simulink model "modelo"  (Simulink 10.0)
settings: Solver=VariableStepAuto  StartTime=0.0  StopTime=stop_time  FixedStep=stop_time/1000  RelTol=1e-5
values from neighbouring files (symbols this model uses):
  alfa1 = 1.4    [erro.m]    (also in natureza.m)
  alfa2 = val(2)    [erro.m]    (also in natureza.m = aux(2))
  delta1 = 3.1    [erro.m]    (also in natureza.m)
  delta2 = -1.5    [erro.m]    (also in natureza.m)
  samp_time = 0.1    [erro.m]    (also in natureza.m = 0.01)
settings Model: Creator=joaotiagoalmeida  LastModifiedBy=joaotiagoalmeida
settings SolverCC: ZeroCrossControl=DisableAll
settings DataIOCC: SaveFormat=Dataset  ReturnWorkspaceOutputs=on
settings OptimizationCC: LifeSpan=auto
settings DebuggingCC: UnderspecifiedInitializationDetection=Simplified  MergeDetectMultiDrivingBlocksExec=error  SFUnexpectedBacktrackingDiag=error  SFNoUnconditionalDefaultTransitionDiag=error  SFExecutionAtInitializationDiag=warning  ArithmeticOperatorsInVariantConditions=error
settings HardwareCC: ProdBitPerPointer=64  ProdBitPerSizeT=64  ProdBitPerPtrDiffT=64  ProdLargestAtomicFloat=Float  ProdIntDivRoundTo=Zero  ProdEndianess=LittleEndian  ProdWordSize=64  ProdHWDeviceType=Intel->x86-64 (Windows64)
settings ModelReferenceCC: PropagateSignalLabelsOutOfModel=on
settings SFSimCC: SimUseLocalCustomCode=on  CustomCodeUndefinedFunction=FilterOut
settings RTWCC: RTWUseLocalCustomCode=on
settings CodeAppCC: StateflowObjectComments=off
settings GRTTargetCC: TargetLangStandard=C99 (ISO)  CombineOutputUpdateFcns=on  GRTInterface=off
settings ConfigComp: CovMetricSettings=dwe  CovHtmlReporting=off  CovSaveCumulativeToWorkspaceVar=off  CovSaveSingleToWorkspaceVar=off

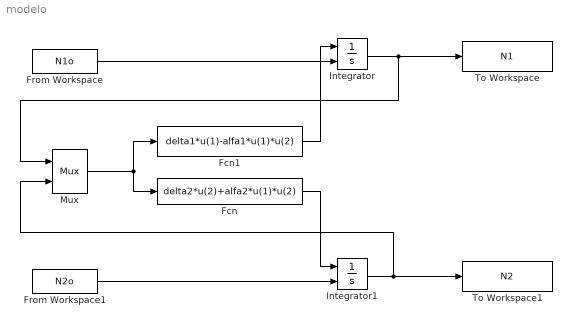
== system modelo ==
  Fcn : Fcn  Expr=delta2*u(2)+alfa2*u(1)*u(2)
  Fcn1 : Fcn  Expr=delta1*u(1)-alfa1*u(1)*u(2)
  From Workspace : FromWorkspace  VariableName=N1o  SampleTime=0
  From Workspace1 : FromWorkspace  VariableName=N2o  SampleTime=0
  Integrator : Integrator  InitialConditionSource=external
  Integrator1 : Integrator  InitialConditionSource=external
  Mux : Mux  Inputs=2
      settings: DisplayOption=signals
  To Workspace : ToWorkspace  VariableName=N1  SampleTime=samp_time
  To Workspace1 : ToWorkspace  VariableName=N2  SampleTime=samp_time
  wires:
  From Workspace/1 -> Integrator/2
  From Workspace1/1 -> Integrator1/2
  Integrator1/1 -> Mux/2, To Workspace1/1
  Integrator/1 -> Mux/1, To Workspace/1
  Fcn/1 -> Integrator1/1
  Fcn1/1 -> Integrator/1
  Mux/1 -> Fcn/1, Fcn1/1
